simulink model "Braking_dynamics_model"  (R2022b)
settings: Solver=VariableStepAuto  StartTime=0.0  StopTime=10.0  RelTol=1e-3
values from neighbouring files (symbols this model uses):
  A = 1.25    [Longitudinal_braking_parameters.m]    (also in Longitudinal_driving_parameters.m)
  a = 1.8    [Longitudinal_braking_parameters.m]    (also in Longitudinal_driving_parameters.m)
  a1 = -1e-5    (= -1e-05)    [Longitudinal_braking_parameters.m]    (also in Longitudinal_driving_parameters.m; Pacejka_lateral_parameters.m)
  a2 = 1.25    [Longitudinal_braking_parameters.m]    (also in Longitudinal_driving_parameters.m; Pacejka_lateral_parameters.m)
  b = L-a    (= 1.7)    [Longitudinal_braking_parameters.m]    (also in Longitudinal_driving_parameters.m)
  B = 4.1576    [Longitudinal_braking_parameters.m]    (also in Longitudinal_driving_parameters.m = 5.7507; Pacejka_lateral_parameters.m = 0.1453)
  C = 1.7180    (= 1.718)    [Longitudinal_braking_parameters.m]    (also in Longitudinal_driving_parameters.m = 1.2421; Pacejka_lateral_parameters.m = 1.5511)
  cd = 0.4    [Longitudinal_braking_parameters.m]    (also in Longitudinal_driving_parameters.m)
  cz = 1    [Longitudinal_braking_parameters.m]    (also in Longitudinal_driving_parameters.m)
  g = 9.81    [Longitudinal_braking_parameters.m]    (also in Longitudinal_driving_parameters.m; Quarter_car_model_parameters.m)
  h = 0.2    [Longitudinal_braking_parameters.m]    (also in Longitudinal_driving_parameters.m)
  Iwheel = 0.9    [Longitudinal_braking_parameters.m]    (also in Longitudinal_driving_parameters.m)
  L = 3.5    [Longitudinal_braking_parameters.m]    (also in Longitudinal_driving_parameters.m)
  m = 850    [Longitudinal_braking_parameters.m]    (also in Longitudinal_driving_parameters.m)
  r = 0.375    [Longitudinal_braking_parameters.m]    (also in Longitudinal_driving_parameters.m)
  rho = 1.225    [Longitudinal_braking_parameters.m]    (also in Longitudinal_driving_parameters.m)
settings Model: Creator=webstert  LastModifiedBy=webstert

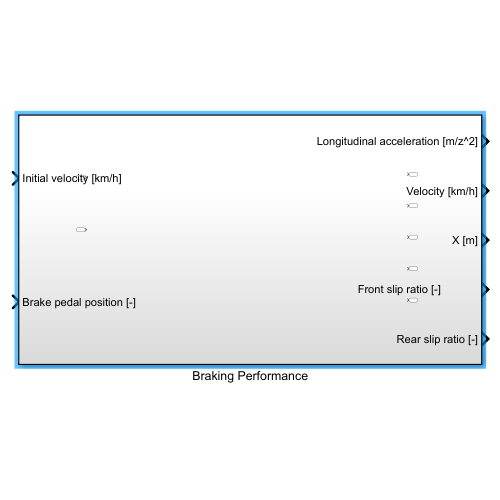
[thumbnail: Simulink's stored preview of the top-level diagram]
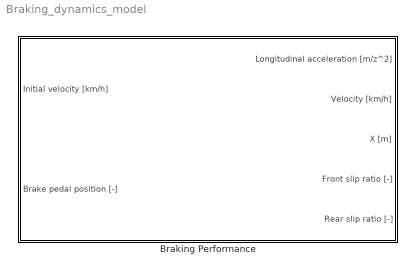
== system Braking_dynamics_model ==
  Braking Performance : Subsystem

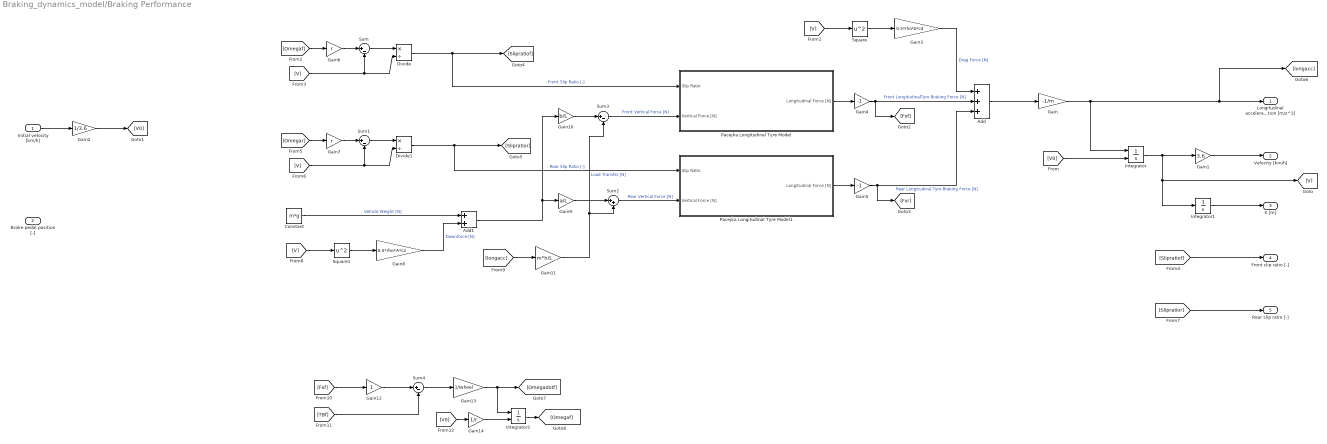
== system Braking_dynamics_model/Braking Performance ==
  Initial velocity [km/h] : Inport
  Brake pedal position [-] : Inport  Port=2
  Add : Sum  Inputs=+++
  Add1 : Sum
  Constant : Constant  Value=m*g
  Divide : Product  Inputs=*/
  Divide1 : Product  Inputs=*/
  Gain : Gain  Gain=-1/m
  Gain1 : Gain  Gain=3.6
  Gain10 : Gain  Gain=b/L
  Gain11 : Gain  Gain=m*h/L
  Gain12 : Gain
  Gain13 : Gain  Gain=1/Iwheel
  Gain14 : Gain  Gain=1/r
  Gain2 : Gain  Gain=1/3.6
  Gain3 : Gain  Gain=0.5*rho*A*cd
  Gain4 : Gain  Gain=-1
  Gain5 : Gain  Gain=-1
  Gain6 : Gain  Gain=r
  Gain7 : Gain  Gain=r
  Gain8 : Gain  Gain=0.5*rho*A*cz
  Gain9 : Gain  Gain=a/L
  Integrator : Integrator  InitialConditionSource=external
  Integrator1 : Integrator
  Integrator2 : Integrator  InitialConditionSource=external
  Pacejka Longitudinal Tyre Model : Subsystem
  Pacejka Longitudinal Tyre Model1 : Subsystem
  Square : Math  Operator=square
  Square1 : Math  Operator=square
  Sum{,1,3..4} (4 alike) : Sum  Inputs=|+-
  Sum2 : Sum  Inputs=|++
  Longitudinal acceleration [m/z^2] : Outport
  Velocity [km/h] : Outport  Port=2
  X [m] : Outport  Port=3
  "Front slip ratio [-]            " : Outport  Port=4
  Rear slip ratio [-] : Outport  Port=5
  wires:
  Add/1 -> Gain/1
  Gain/1 -> Integrator/1, [longacc], Longitudinal acceleration [m/z^2]/1
  Gain1/1 -> Velocity [km/h]/1
  Integrator/1 -> Gain1/1, [V], Integrator1/1
  Integrator1/1 -> X [m]/1
  Gain2/1 -> [V0]
  Initial velocity [km/h]/1 -> Gain2/1
  [V0] -> Integrator/2
  [V] -> Square/1
  Square/1 -> Gain3/1
  Gain3/1 -> Add/1  "Drag Force [N]"
  Pacejka Longitudinal Tyre Model/1(Longitudinal Force [N]) -> Gain4/1
  Gain4/1 -> [Fxf], Add/2  "Front LongitudinalTyre Braking Force [N]"
  Pacejka Longitudinal Tyre Model1/1(Longitudinal Force [N]) -> Gain5/1
  Gain5/1 -> [Fxr], Add/3  "Rear Longitudinal Tyre Braking Force [N]"
  [Omegaf] -> Gain6/1
  Gain6/1 -> Sum/1
  [V] -> Sum/2, Divide/2
  Sum/1 -> Divide/1
  Divide/1 -> [Slipratiof], Pacejka Longitudinal Tyre Model/1(Slip Ratio)  "Front Slip Ratio [-]"
  [Slipratiof] -> "Front slip ratio [-]            "/1
  Divide1/1 -> Pacejka Longitudinal Tyre Model1/1(Slip Ratio), [Slipratior]  "Rear Slip Ratio [-]"
  Sum1/1 -> Divide1/1
  [V] -> Divide1/2, Sum1/2
  Gain7/1 -> Sum1/1
  [Omegar] -> Gain7/1
  [Slipratior] -> Rear slip ratio [-]/1
  Square1/1 -> Gain8/1
  Gain8/1 -> Add1/2  "Downforce [N]"
  [V] -> Square1/1
  Constant/1 -> Add1/1  "Vehicle Weight [N]"
  Add1/1 -> Gain9/1, Gain10/1
  Sum3/1 -> Pacejka Longitudinal Tyre Model/2(Vertical Force [N])  "Front Vertical Force [N]"
  Gain9/1 -> Sum2/1
  Sum2/1 -> Pacejka Longitudinal Tyre Model1/2(Vertical Force [N])  "Rear Vertical Force [N]"
  Gain10/1 -> Sum3/1
  [longacc] -> Gain11/1
  Gain11/1 -> Sum2/2, Sum3/2  "Load Transfer [N]"
  [Fxf] -> Gain12/1
  Gain12/1 -> Sum4/1
  [TBf] -> Sum4/2
  Sum4/1 -> Gain13/1
  Gain13/1 -> Integrator2/1, [Omegadotf]
  Integrator2/1 -> [Omegaf]
  [V0] -> Gain14/1
  Gain14/1 -> Integrator2/2

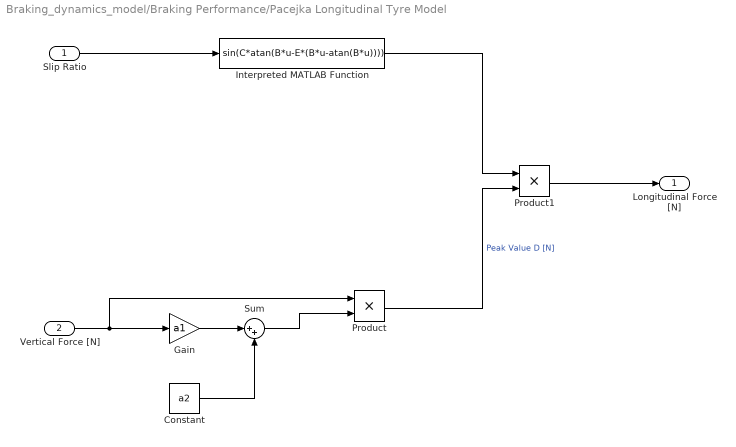
== system Braking_dynamics_model/Braking Performance/Pacejka Longitudinal Tyre Model ==
  Slip Ratio : Inport
  Vertical Force [N] : Inport  Port=2
  Constant : Constant  Value=a2
  Gain : Gain  Gain=a1
  Interpreted MATLAB Function : MATLABFcn  MATLABFcn=sin(C*atan(B*u-E*(B*u-atan(B*u))))
  Product : Product
  Product1 : Product
  Sum : Sum  Inputs=|++
  Longitudinal Force [N] : Outport
  wires:
  Vertical Force [N]/1 -> Product/1, Gain/1
  Constant/1 -> Sum/2
  Gain/1 -> Sum/1
  Sum/1 -> Product/2
  Product/1 -> Product1/2  "Peak Value D [N]"
  Slip Ratio/1 -> Interpreted MATLAB Function/1
  Interpreted MATLAB Function/1 -> Product1/1
  Product1/1 -> Longitudinal Force [N]/1

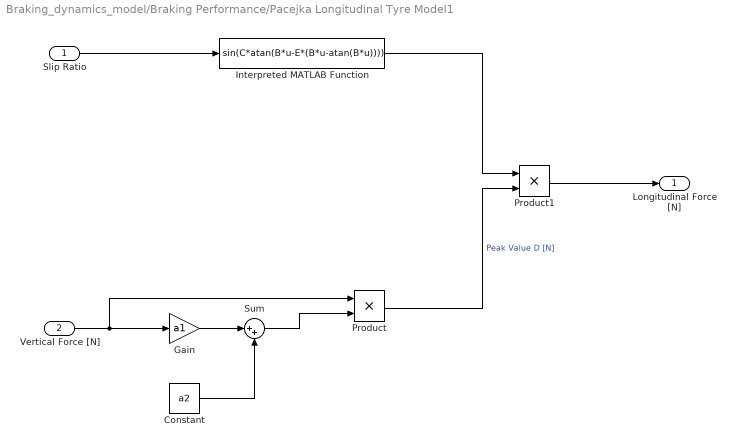
== system Braking_dynamics_model/Braking Performance/Pacejka Longitudinal Tyre Model1 ==
  Slip Ratio : Inport
  Vertical Force [N] : Inport  Port=2
  Constant : Constant  Value=a2
  Gain : Gain  Gain=a1
  Interpreted MATLAB Function : MATLABFcn  MATLABFcn=sin(C*atan(B*u-E*(B*u-atan(B*u))))
  Product : Product
  Product1 : Product
  Sum : Sum  Inputs=|++
  Longitudinal Force [N] : Outport
  wires:
  Product1/1 -> Longitudinal Force [N]/1
  Interpreted MATLAB Function/1 -> Product1/1
  Slip Ratio/1 -> Interpreted MATLAB Function/1
  Product/1 -> Product1/2  "Peak Value D [N]"
  Sum/1 -> Product/2
  Gain/1 -> Sum/1
  Constant/1 -> Sum/2
  Vertical Force [N]/1 -> Gain/1, Product/1
